simulink subsystem "kls_motor_interface"  (R2025b)
settings: Solver=VariableStepAuto  StartTime=0.0  StopTime=10.0  RelTol=1e-3
libraries: simulink x1, slpidlib x1
settings Model: Creator=orang  LastModifiedBy=erik

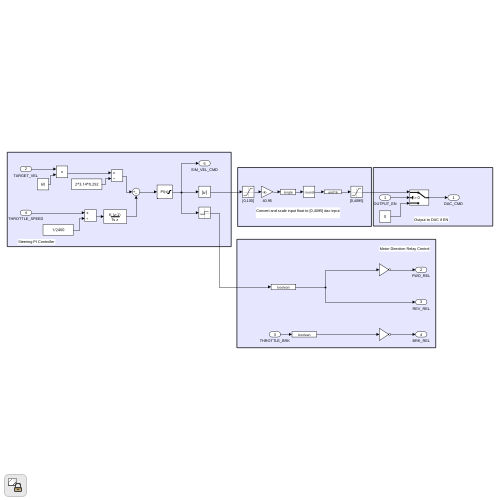
[thumbnail: Simulink's stored preview of the top-level diagram]
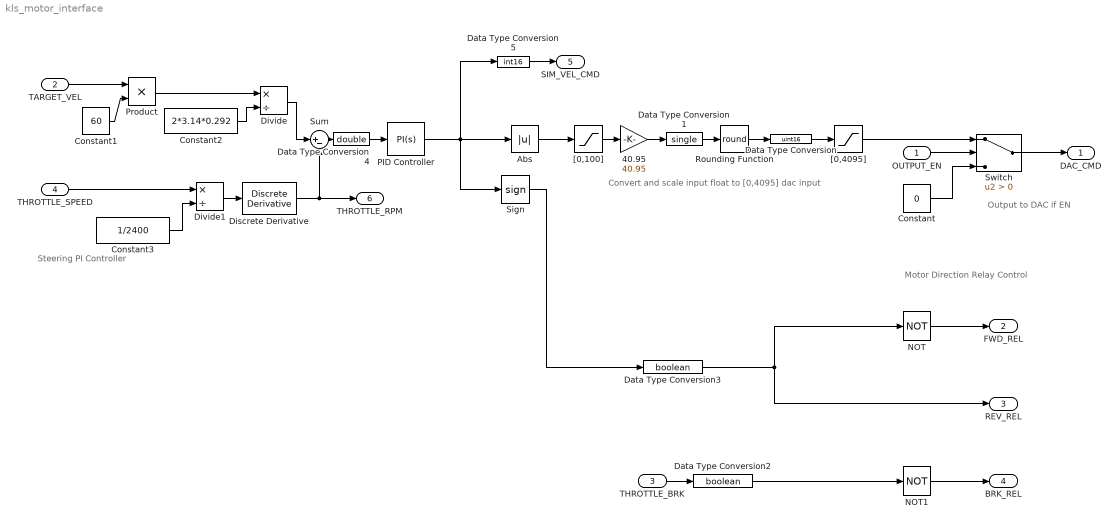
== system kls_motor_interface ==
  note: Steering PI Controller
  note: Motor Direction Relay Control
  note: Output to DAC if EN
  note: Convert and scale input float to [0,4095] dac input
  OUTPUT_EN : Inport  OutDataTypeStr=boolean
  TARGET_VEL : Inport  Port=2
  THROTTLE_BRK : Inport  Port=3
  THROTTLE_SPEED : Inport  Port=4
  40.95 : Gain  Gain=40.95  OutDataTypeStr=uint16
  Abs : Abs  SaturateOnIntegerOverflow=off
  Constant : Constant  Value=0
  Constant1 : Constant  Value=60
  Constant2 : Constant  Value=2*3.14*0.292
  Constant3 : Constant  Value=1/2400
  Data Type Conversion : DataTypeConversion  OutDataTypeStr=uint16  SaturateOnIntegerOverflow=off  RndMeth=Floor
  Data Type Conversion1 : DataTypeConversion  OutDataTypeStr=single  SaturateOnIntegerOverflow=off  RndMeth=Floor
  Data Type Conversion2 : DataTypeConversion  OutDataTypeStr=boolean  SaturateOnIntegerOverflow=off  RndMeth=Floor
  Data Type Conversion3 : DataTypeConversion  OutDataTypeStr=boolean  SaturateOnIntegerOverflow=off  RndMeth=Floor
  Data Type Conversion4 : DataTypeConversion  OutDataTypeStr=double  SaturateOnIntegerOverflow=off  RndMeth=Floor
  Data Type Conversion5 : DataTypeConversion  OutDataTypeStr=int16  SaturateOnIntegerOverflow=off  RndMeth=Floor
  Discrete Derivative : simulink/Quick Insert/Discrete/Discrete Derivative  gainval=1.0  ICPrevScaledInput=0.0  OutMin=[]  OutMax=[]  OutDataType=fixdt(1, 16)  OutScaling=2^-10  DoSatur=off
  Divide : Product  Inputs=*/
  Divide1 : Product  Inputs=*/
  NOT : Logic  Operator=NOT  IconShape=distinctive  AllPortsSameDT=off  OutDataTypeStr=boolean
  NOT1 : Logic  Operator=NOT  IconShape=distinctive  AllPortsSameDT=off  OutDataTypeStr=boolean
  PID Controller : slpidlib/PID Controller  Controller=PI  Form=Parallel  TimeDomain=Continuous-time  UseExternalTs=off  SampleTime=-1  IntegratorMethod=Forward Euler  FilterMethod=Forward Euler  ControllerParametersSource=internal  P=1  I=1  UseKiTs=on  D=0  UseExternalDerivativeSource=off  N=100  UseFilter=on  TunerSelectOption=Transfer Function Based (PID Tuner App)  InitialConditionSource=internal  InitialConditionForIntegrator=0  InitialConditionForFilter=0  DifferentiatorICPrevScaledInput=0  ExternalReset=none  TrackingMode=off  Kt=1  LimitOutput=on  SatLimitsSource=internal  UpperSaturationLimit=100  LowerSaturationLimit=-100  LinearizeAsGain=on  AntiWindupMode=back-calculation  Kb=1  LimitIntegrator=off  UpperIntegratorSaturationLimit=inf  LowerIntegratorSaturationLimit=-inf  POutMin=[]  POutMax=[]  IOutMin=[]  IOutMax=[]  DOutMin=[]  DOutMax=[]  NOutMin=[]  NOutMax=[]  SumOutMin=[]  SumOutMax=[]  SaturationOutMin=[]  SaturationOutMax=[]  PParamMin=[]  PParamMax=[]  IParamMin=[]  IParamMax=[]  DParamMin=[]  DParamMax=[]  NParamMin=[]  NParamMax=[]  KbParamMin=[]  KbParamMax=[]  KtParamMin=[]  KtParamMax=[]  KbOutMin=[]  KbOutMax=[]  KtOutMin=[]  KtOutMax=[]  IntegratorOutMin=[]  IntegratorOutMax=[]  FilterOutMin=[]  FilterOutMax=[]  SumI1OutMin=[]  SumI1OutMax=[]  SumI2OutMin=[]  SumI2OutMax=[]  SumI3OutMin=[]  SumI3OutMax=[]  SumI4OutMin=[]  SumI4OutMax=[]  SumDOutMin=[]  SumDOutMax=[]  DifferentiatorOutMin=[]  DifferentiatorOutMax=[]  FilterDiffOutCoefMin=[]  FilterDiffOutCoefMax=[]  ReciprocalOutMin=[]  ReciprocalOutMax=[]  SumDenOutMin=[]  SumDenOutMax=[]  SumNumOutMin=[]  SumNumOutMax=[]  DivideOutMin=[]  DivideOutMax=[]  UdiffTsProdOutMin=[]  UdiffTsProdOutMax=[]  NTsProdOutMin=[]  NTsProdOutMax=[]  UintegralTsProdOutMin=[]  UintegralTsProdOutMax=[]  UngainTsProdOutMin=[]  UngainTsProdOutMax=[]  ClampingZeroOutDataTypeStr=Inherit: Inherit via back propagation  ClampingZeroOutMin=[]  ClampingZeroOutMax=[]  FilterDenConstantOutDataTypeStr=Inherit: Inherit via back propagation  FilterDenConstantOutMin=[]  FilterDenConstantOutMax=[]  PCopyOutDataTypeStr=Inherit: Inherit via back propagation  PCopyOutMin=[]  PCopyOutMax=[]  NCopyOutDataTypeStr=Inherit: Inherit via back propagation  NCopyOutMin=[]  NCopyOutMax=[]  IntegratorContinuousStateAttributes=''  IntegratorStateMustResolveToSignalObject=off  IntegratorRTWStateStorageClass=Auto  FilterContinuousStateAttributes=''  FilterStateMustResolveToSignalObject=off  FilterRTWStateStorageClass=Auto  ParallelPVariant=InternalParameters  IdealPVariant=Disabled  IVariant=InternalParameters  DVariant=Disabled  IntegratorVariant=Continuous  SatVariant=Enabled  AWVariant=BackCalculation  PCopyVariant=Disabled  TRVariant=Disabled  FdbkBlocksVariant=Forward  IdealPFdbkVariant=Disabled  SatFdbkVariant=Disabled  DerivativeFilterVariant=Disabled  NVariant=Disabled  NCopyVariant=Disabled_SignalSpec  FilterICVariant=Disabled  IntegratorICVariant=InternalICs  ExternalResetVariant=Disabled  TRSumVariant=Passthrough  SumFdbkVariant=Disabled  SumVariant=Sum_PI  TsampFilterVariant=InternalTs  TsampNgainVariant=Passthrough  TsampIntegralVariant=Disabled_SignalSpec  ExternalSaturationOutDataTypeStr=Inherit: Same as second input  DerivativeSourceVariant=Disabled  PreIntVariant=InternalPreInt
  Product : Product
  Rounding Function : Rounding  Operator=round
  Sign : Signum
  Sum : Sum  Inputs=|+-
  Switch : Switch  Criteria=u2 > Threshold  OutDataTypeStr=uint16  SaturateOnIntegerOverflow=off  InputSameDT=off
  "[0,100]" : Saturate  UpperLimit=100  LowerLimit=0
  "[0,4095]" : Saturate  UpperLimit=4095  LowerLimit=0
  DAC_CMD : Outport
  FWD_REL : Outport  Port=2
  REV_REL : Outport  Port=3
  BRK_REL : Outport  Port=4
  SIM_VEL_CMD : Outport  Port=5
  THROTTLE_RPM : Outport  Port=6
  wires:
  Rounding Function/1 -> Data Type Conversion/1
  Data Type Conversion/1 -> "[0,4095]"/1
  "[0,100]"/1 -> 40.95/1
  40.95/1 -> Data Type Conversion1/1
  OUTPUT_EN/1 -> Switch/2
  Constant/1 -> Switch/3
  Data Type Conversion1/1 -> Rounding Function/1
  THROTTLE_BRK/1 -> Data Type Conversion2/1
  Data Type Conversion2/1 -> NOT1/1
  Data Type Conversion3/1 -> NOT/1, REV_REL/1
  NOT/1 -> FWD_REL/1
  NOT1/1 -> BRK_REL/1
  Switch/1 -> DAC_CMD/1
  "[0,4095]"/1 -> Switch/1
  TARGET_VEL/1 -> Product/1
  Constant1/1 -> Product/2
  Constant2/1 -> Divide/2
  Product/1 -> Divide/1
  Discrete Derivative/1 -> Sum/2, THROTTLE_RPM/1
  Divide/1 -> Sum/1
  Divide1/1 -> Discrete Derivative/1
  THROTTLE_SPEED/1 -> Divide1/1
  Constant3/1 -> Divide1/2
  Abs/1 -> "[0,100]"/1
  PID Controller/1 -> Sign/1, Abs/1, Data Type Conversion5/1
  Sign/1 -> Data Type Conversion3/1
  Sum/1 -> Data Type Conversion4/1
  Data Type Conversion4/1 -> PID Controller/1
  Data Type Conversion5/1 -> SIM_VEL_CMD/1
